simulink model "playground"  (R2019b)
settings: Solver=VariableStepAuto  StartTime=0.0  StopTime=0.01  RelTol=1e-3
values from neighbouring files (symbols this model uses):
  C = pid(Kp, Ki, Kd, 0)    [AHHHHHH.m]    (also in currentTester.m = 7.5e-07; manPID.m = pid(Kp, Ki, Kd); part2.m = pid(Kp, Ki, Kd); take2.m = 7.5e-07)
  fs = 50*10^3    (= 50000)    [AHHHHHH.m]    (also in currentTester.m; manPID.m; part2.m; take2.m)
  L = 1.7e-3    (= 0.0017)    [AHHHHHH.m]    (also in currentTester.m; manPID.m; part2.m; take2.m)
  RC = 0.03    [AHHHHHH.m]    (also in currentTester.m; manPID.m; part2.m; take2.m)
  RL = 0.08    [AHHHHHH.m]    (also in currentTester.m; manPID.m; part2.m; take2.m)
  RLoad = 100    [AHHHHHH.m]    (also in currentTester.m = rRange(it); manPID.m = 100,000; part2.m; take2.m)
  Vin = 24    [AHHHHHH.m]    (also in currentTester.m; manPID.m; part2.m; take2.m)
  vinNoise = 0    [currentTester.m]
  Vref = 18    [AHHHHHH.m]    (also in currentTester.m; manPID.m; part2.m; take2.m)
libraries: simulink x1, powerlib_meascontrol x1
settings Model: Creator=russty  LastModifiedBy=TimRo
settings SolverCC: ZeroCrossAlgorithm=Adaptive
settings DebuggingCC: MaskedZcDiagnostic=none  IgnoredZcDiagnostic=none

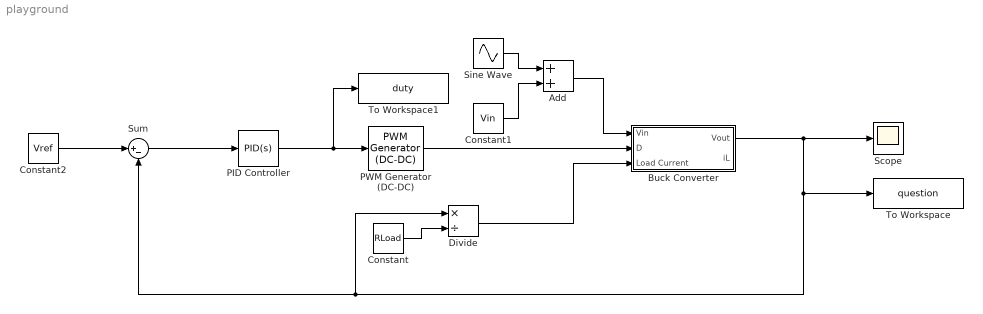
== system playground ==
  Add : Sum
  Buck Converter : Subsystem
  Constant : Constant  Value=RLoad
  Constant1 : Constant  Value=Vin
  Constant2 : Constant  Value=Vref
  Divide : Product  Inputs=*/
  PID Controller : simulink/Continuous/PID Controller  Controller=PID  Form=Parallel  TimeDomain=Continuous-time  SampleTime=-1  IntegratorMethod=Forward Euler  FilterMethod=Forward Euler  ControllerParametersSource=internal  P=-119544800000000000  I=171621102000000008192  D=7300000000000  UseFilter=on  N=100  TunerSelectOption=Transfer Function Based (PID Tuner App)  InitialConditionSource=internal  InitialConditionForIntegrator=0  InitialConditionForFilter=0  DifferentiatorICPrevScaledInput=0  ExternalReset=none  TrackingMode=off  Kt=1  LimitOutput=off  UpperSaturationLimit=inf  LowerSaturationLimit=-inf  LinearizeAsGain=on  AntiWindupMode=none  Kb=1  POutMin=[]  POutMax=[]  IOutMin=[]  IOutMax=[]  DOutMin=[]  DOutMax=[]  NOutMin=[]  NOutMax=[]  SumOutMin=[]  SumOutMax=[]  SaturationOutMin=[]  SaturationOutMax=[]  PParamMin=[]  PParamMax=[]  IParamMin=[]  IParamMax=[]  DParamMin=[]  DParamMax=[]  NParamMin=[]  NParamMax=[]  KbParamMin=[]  KbParamMax=[]  KtParamMin=[]  KtParamMax=[]  KbOutMin=[]  KbOutMax=[]  KtOutMin=[]  KtOutMax=[]  IntegratorOutMin=[]  IntegratorOutMax=[]  FilterOutMin=[]  FilterOutMax=[]  SumI1OutMin=[]  SumI1OutMax=[]  SumI2OutMin=[]  SumI2OutMax=[]  SumI3OutMin=[]  SumI3OutMax=[]  SumI4OutMin=[]  SumI4OutMax=[]  SumDOutMin=[]  SumDOutMax=[]  DifferentiatorOutMin=[]  DifferentiatorOutMax=[]  FilterDiffOutCoefMin=[]  FilterDiffOutCoefMax=[]  ReciprocalOutMin=[]  ReciprocalOutMax=[]  SumDenOutMin=[]  SumDenOutMax=[]  SumNumOutMin=[]  SumNumOutMax=[]  DivideOutMin=[]  DivideOutMax=[]  IntegratorContinuousStateAttributes=''  IntegratorStateMustResolveToSignalObject=off  IntegratorRTWStateStorageClass=Auto  FilterContinuousStateAttributes=''  FilterStateMustResolveToSignalObject=off  FilterRTWStateStorageClass=Auto  ParallelPVariant=InternalParameters  IdealPVariant=Disabled  IVariant=InternalParameters  DVariant=InternalParameters  IntegratorVariant=Continuous  SatVariant=Disabled  AWVariant=Passthrough  PCopyVariant=Disabled  TRVariant=Disabled  FdbkBlocksVariant=Forward  IdealPFdbkVariant=Disabled  SatFdbkVariant=Disabled  DerivativeFilterVariant=ContFilter  NVariant=InternalParameters  NCopyVariant=Disabled  FilterICVariant=InternalICsFilter  IntegratorICVariant=InternalICs  ExternalResetVariant=Disabled  TRSumVariant=Passthrough  SumFdbkVariant=Disabled  SumVariant=Sum_PID
  PWM Generator (DC-DC) : powerlib_meascontrol/Pulse & Signal Generators/PWM Generator (DC-DC)  Fsw=1/fs  Ts=0
      settings: SourceProductName=Simscape Electrical
  Scope : Scope
  Sine Wave : Sin  Amplitude=vinNoise  Frequency=120*pi()  SampleTime=0
  Sum : Sum  Inputs=|+-
  To Workspace : ToWorkspace  VariableName=question  SaveFormat=Timeseries  SampleTime=-1
  To Workspace1 : ToWorkspace  VariableName=duty  SaveFormat=Timeseries  SampleTime=-1
  wires:
  Divide/1 -> Buck Converter/3(Load Current)
  Constant/1 -> Divide/2
  Sum/1 -> PID Controller/1
  Constant2/1 -> Sum/1
  Buck Converter/1(Vout) -> Scope/1, To Workspace/1, Sum/2, Divide/1
  PID Controller/1 -> PWM Generator (DC-DC)/1, To Workspace1/1
  Sine Wave/1 -> Add/1
  Constant1/1 -> Add/2
  Add/1 -> Buck Converter/1(Vin)
  PWM Generator (DC-DC)/1 -> Buck Converter/2(D)

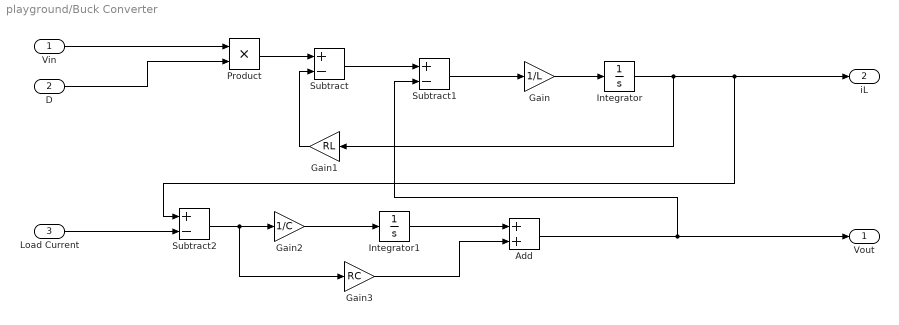
== system playground/Buck Converter ==
  Vin : Inport
  D : Inport  Port=2
  Load Current : Inport  Port=3
  Add : Sum
  Gain : Gain  Gain=1/L
  Gain1 : Gain  Gain=RL
  Gain2 : Gain  Gain=1/C
  Gain3 : Gain  Gain=RC
  Integrator : Integrator
  Integrator1 : Integrator
  Product : Product
  Subtract : Sum  Inputs=+-
  Subtract1 : Sum  Inputs=+-
  Subtract2 : Sum  Inputs=+-
  Vout : Outport
  iL : Outport  Port=2
  wires:
  Vin/1 -> Product/1
  D/1 -> Product/2
  Product/1 -> Subtract/1
  Subtract/1 -> Subtract1/1
  Subtract1/1 -> Gain/1
  Gain/1 -> Integrator/1
  Integrator/1 -> Gain1/1, Subtract2/1, iL/1
  Gain1/1 -> Subtract/2
  Load Current/1 -> Subtract2/2
  Subtract2/1 -> Gain3/1, Gain2/1
  Gain2/1 -> Integrator1/1
  Integrator1/1 -> Add/1
  Gain3/1 -> Add/2
  Add/1 -> Subtract1/2, Vout/1
